simulink library "TQD_lib"  (Simulink 7.5)
settings: Solver=ode45  StartTime=0.0  StopTime=10.0  RelTol=1e-3
values from neighbouring files (symbols this model uses):
  pTQD_bool_ZeroCrossingEnabl_C = Simulink.Parameter    [TQD_par.m]
  pTQD_Nm_HiTqRecoverThd_C = Simulink.Parameter    [TQD_par.m]
  pTQD_Nm_MaxPrimTMTrq_C = Simulink.Parameter    [TQD_par.m]
  pTQD_Nm_MaxSecTMTrq_C = Simulink.Parameter    [TQD_par.m]
  pTQD_Nm_MinPrimTMTrq_C = Simulink.Parameter    [TQD_par.m]
  pTQD_Nm_MinSecTMTrq_C = Simulink.Parameter    [TQD_par.m]
  pTQD_Nm_TMTrqMinus_C = Simulink.Parameter    [TQD_par.m]
  pTQD_Nm_TqLowrCrossHiThd_C = Simulink.Parameter    [TQD_par.m]
  pTQD_Nm_TqLowrCrossThd_C = Simulink.Parameter    [TQD_par.m]
  pTQD_Nm_TqUpprCrossHiThd_C = Simulink.Parameter    [TQD_par.m]
  pTQD_Nm_TqUpprCrossThd_C = Simulink.Parameter    [TQD_par.m]
  pTQD_Nmps_TrqLoRateLimit_C = Simulink.Parameter    [TQD_par.m]
  pTQD_Nmps_TrqUpRateLimit_C = Simulink.Parameter    [TQD_par.m]
  pTQD_r_DrvNearZeroFilterFac_C = Simulink.Parameter    [TQD_par.m]
  pTQD_r_DrvZeroCrsFilterFac_C = Simulink.Parameter    [TQD_par.m]
  pTQD_r_NormalFilterFac_C = Simulink.Parameter    [TQD_par.m]
  pTQD_rpm_TMZeroSpd_C = Simulink.Parameter    [TQD_par.m]
  pTQD_s_TqZeroCrossTiout_C = Simulink.Parameter    [TQD_par.m]
undefined symbols (not defined in the file or in its folder): p_single_Minus_M, p_single_Plus_M, p_single_Zero_M, p_st_DrvModeFlg_C
libraries: BaseOperationLib_Browser x95, simulink x1
settings Model: Creator=wuaibin  LastModifiedBy=wuaibin

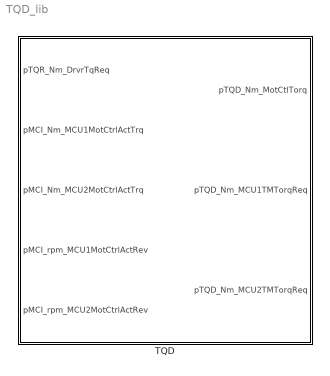
== system TQD_lib ==
  TQD : Subsystem  TreatAsAtomicUnit=on

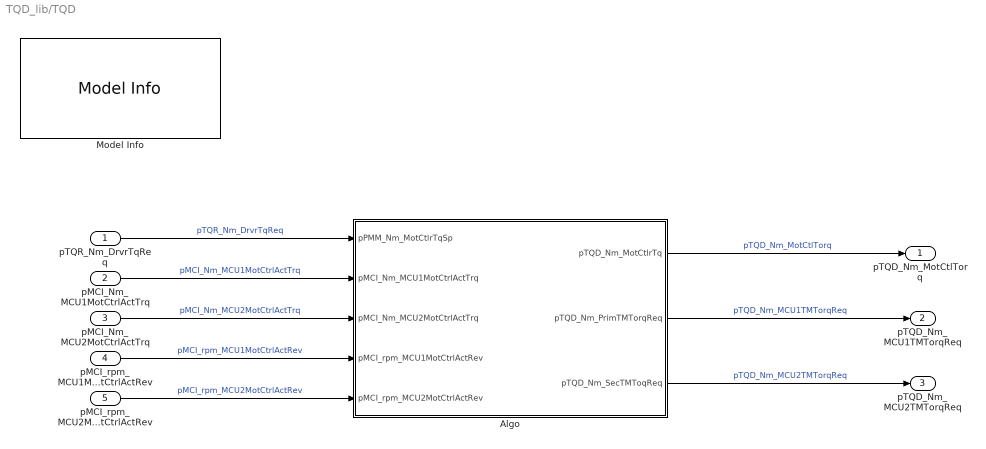
== system TQD_lib/TQD ==
  pTQR_Nm_DrvrTqReq : Inport  OutDataType=fixdt(1, 16)  OutScaling=2^0
  pMCI_Nm_MCU1MotCtrlActTrq : Inport  Port=2
  pMCI_Nm_MCU2MotCtrlActTrq : Inport  Port=3
  pMCI_rpm_MCU1MotCtrlActRev : Inport  Port=4  OutDataType=fixdt(1, 16)  OutScaling=2^0
  pMCI_rpm_MCU2MotCtrlActRev : Inport  Port=5  OutDataType=fixdt(1, 16)  OutScaling=2^0
  Algo : Subsystem
  Model Info : simulink/Model-Wide Utilities/Model Info  SystemSampleTime=-1  InitialBlockCM=None  BlockCM=None  Frame=on  DisplayStringWithTags=Model Info\nCreated: %<Created>\nCreator: %<Creator>  HorizontalTextAlignment=Center  LeftAlignmentValue=0.5  SourceBlockDiagram=HQEV_HCU  TagMaxNumber=20
  pTQD_Nm_MotCtlTorq : Outport  OutDataType=fixdt(1, 16)  OutScaling=2^0
  pTQD_Nm_MCU1TMTorqReq : Outport  Port=2
  pTQD_Nm_MCU2TMTorqReq : Outport  Port=3
  wires:
  pMCI_rpm_MCU2MotCtrlActRev/1 -> Algo/5(pMCI_rpm_MCU2MotCtrlActRev)  "pMCI_rpm_MCU2MotCtrlActRev"
  pMCI_rpm_MCU1MotCtrlActRev/1 -> Algo/4(pMCI_rpm_MCU1MotCtrlActRev)  "pMCI_rpm_MCU1MotCtrlActRev"
  pTQR_Nm_DrvrTqReq/1 -> Algo/1(pPMM_Nm_MotCtlrTqSp)  "pTQR_Nm_DrvrTqReq"
  pMCI_Nm_MCU1MotCtrlActTrq/1 -> Algo/2(pMCI_Nm_MCU1MotCtrlActTrq)  "pMCI_Nm_MCU1MotCtrlActTrq"
  pMCI_Nm_MCU2MotCtrlActTrq/1 -> Algo/3(pMCI_Nm_MCU2MotCtrlActTrq)  "pMCI_Nm_MCU2MotCtrlActTrq"
  Algo/1(pTQD_Nm_MotCtlrTq) -> pTQD_Nm_MotCtlTorq/1  "pTQD_Nm_MotCtlTorq"
  Algo/2(pTQD_Nm_PrimTMTorqReq) -> pTQD_Nm_MCU1TMTorqReq/1  "pTQD_Nm_MCU1TMTorqReq"
  Algo/3(pTQD_Nm_SecTMToqReq) -> pTQD_Nm_MCU2TMTorqReq/1  "pTQD_Nm_MCU2TMTorqReq"

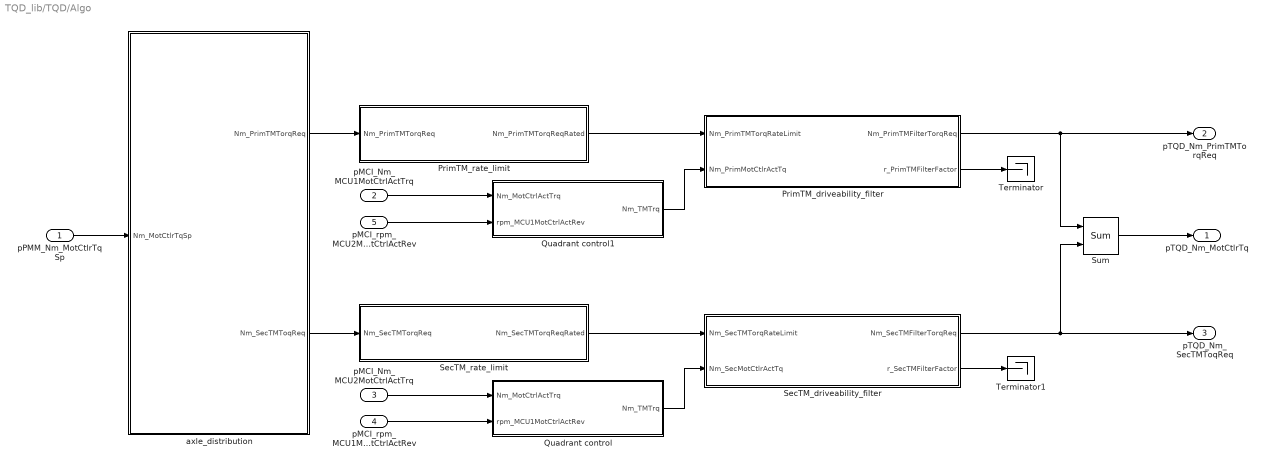
== system TQD_lib/TQD/Algo ==
  pPMM_Nm_MotCtlrTqSp : Inport  OutDataType=fixdt(1, 16)  OutScaling=2^0
  pMCI_Nm_MCU1MotCtrlActTrq : Inport  Port=2
  pMCI_Nm_MCU2MotCtrlActTrq : Inport  Port=3
  pMCI_rpm_MCU1MotCtrlActRev : Inport  Port=4  OutDataType=fixdt(1, 16)  OutScaling=2^0
  pMCI_rpm_MCU2MotCtrlActRev : Inport  Port=5  OutDataType=fixdt(1, 16)  OutScaling=2^0
  PrimTM_driveability_filter : Subsystem
  PrimTM_rate_limit : Subsystem
  Quadrant control : Subsystem
  Quadrant control1 : Subsystem
  SecTM_driveability_filter : Subsystem
  SecTM_rate_limit : Subsystem
  Sum : BaseOperationLib_Browser/Math Operations Changed/Sum  Inputs=++  InputSameDT=on  OutMin=[]  OutMax=[]  OutDataType=fixdt(1, 16)  OutScaling=2^0  SaturateOnIntegerOverflow=on
  Terminator : Terminator
  Terminator1 : Terminator
  axle_distribution : Subsystem
  pTQD_Nm_MotCtlrTq : Outport  OutDataType=fixdt(1, 16)  OutScaling=2^0
  pTQD_Nm_PrimTMTorqReq : Outport  Port=2
  pTQD_Nm_SecTMToqReq : Outport  Port=3
  wires:
  pMCI_rpm_MCU2MotCtrlActRev/1 -> Quadrant control1/2(rpm_MCU1MotCtrlActRev)
  pMCI_Nm_MCU1MotCtrlActTrq/1 -> Quadrant control1/1(Nm_MotCtrlActTrq)
  Quadrant control1/1(Nm_TMTrq) -> PrimTM_driveability_filter/2(Nm_PrimMotCtlrActTq)
  Quadrant control/1(Nm_TMTrq) -> SecTM_driveability_filter/2(Nm_SecMotCtlrActTq)
  pMCI_rpm_MCU1MotCtrlActRev/1 -> Quadrant control/2(rpm_MCU1MotCtrlActRev)
  pMCI_Nm_MCU2MotCtrlActTrq/1 -> Quadrant control/1(Nm_MotCtrlActTrq)
  SecTM_driveability_filter/1(Nm_SecTMFilterTorqReq) -> Sum/2, pTQD_Nm_SecTMToqReq/1
  PrimTM_driveability_filter/1(Nm_PrimTMFilterTorqReq) -> Sum/1, pTQD_Nm_PrimTMTorqReq/1
  pPMM_Nm_MotCtlrTqSp/1 -> axle_distribution/1(Nm_MotCtlrTqSp)
  Sum/1 -> pTQD_Nm_MotCtlrTq/1
  axle_distribution/1(Nm_PrimTMTorqReq) -> PrimTM_rate_limit/1(Nm_PrimTMTorqReq)
  PrimTM_rate_limit/1(Nm_PrimTMTorqReqRated) -> PrimTM_driveability_filter/1(Nm_PrimTMTorqRateLimit)
  SecTM_rate_limit/1(Nm_SecTMTorqReqRated) -> SecTM_driveability_filter/1(Nm_SecTMTorqRateLimit)
  axle_distribution/2(Nm_SecTMToqReq) -> SecTM_rate_limit/1(Nm_SecTMTorqReq)
  PrimTM_driveability_filter/2(r_PrimTMFilterFactor) -> Terminator/1
  SecTM_driveability_filter/2(r_SecTMFilterFactor) -> Terminator1/1

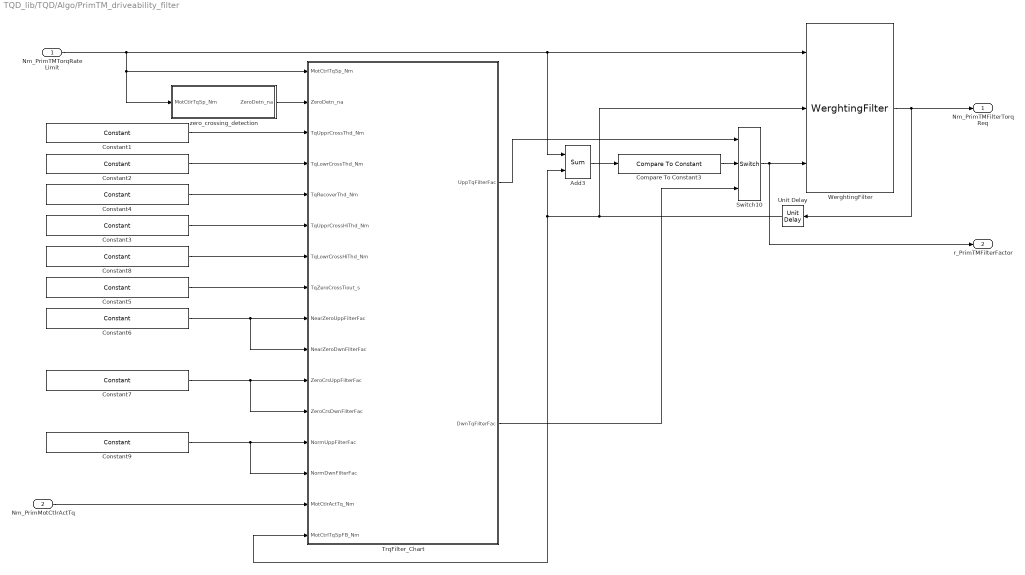
== system TQD_lib/TQD/Algo/PrimTM_driveability_filter ==
  Nm_PrimTMTorqRateLimit : Inport
  Nm_PrimMotCtlrActTq : Inport  Port=2
  Add3 : BaseOperationLib_Browser/Math Operations Changed/Sum  Inputs=+-  OutMin=[]  OutMax=[]  OutDataType=fixdt(1, 16)  OutScaling=2^0
  Compare To Constant3 : BaseOperationLib_Browser/Logic Operations Changed/Compare To Constant  SystemSampleTime=-1  relop=>=  const=p_single_Zero_M
  Constant1 : BaseOperationLib_Browser/Sources&Sinks/Constant  Value=pTQD_Nm_TqUpprCrossThd_C  OutMin=[]  OutMax=[]  OutDataType=fixdt(1, 16)  ConRadixGroup=Use specified scaling  OutScaling=2^0  OutDataTypeStr=Inherit: Inherit from 'Constant value'
  Constant2 : BaseOperationLib_Browser/Sources&Sinks/Constant  Value=pTQD_Nm_TqLowrCrossThd_C  OutMin=[]  OutMax=[]  OutDataType=fixdt(1, 16)  ConRadixGroup=Use specified scaling  OutScaling=2^0  OutDataTypeStr=Inherit: Inherit from 'Constant value'
  Constant3 : BaseOperationLib_Browser/Sources&Sinks/Constant  Value=pTQD_Nm_TqUpprCrossHiThd_C  OutMin=[]  OutMax=[]  OutDataType=fixdt(1, 16)  ConRadixGroup=Use specified scaling  OutScaling=2^0  OutDataTypeStr=Inherit: Inherit from 'Constant value'
  Constant4 : BaseOperationLib_Browser/Sources&Sinks/Constant  Value=pTQD_Nm_HiTqRecoverThd_C  OutMin=[]  OutMax=[]  OutDataType=fixdt(1, 16)  ConRadixGroup=Use specified scaling  OutScaling=2^0  OutDataTypeStr=Inherit: Inherit from 'Constant value'
  Constant5 : BaseOperationLib_Browser/Sources&Sinks/Constant  Value=pTQD_s_TqZeroCrossTiout_C  OutMin=[]  OutMax=[]  OutDataType=fixdt(1, 16)  ConRadixGroup=Use specified scaling  OutScaling=2^0  OutDataTypeStr=Inherit: Inherit from 'Constant value'
  Constant6 : BaseOperationLib_Browser/Sources&Sinks/Constant  Value=pTQD_r_DrvNearZeroFilterFac_C  OutMin=[]  OutMax=[]  OutDataType=fixdt(1, 16)  ConRadixGroup=Use specified scaling  OutScaling=2^0  OutDataTypeStr=Inherit: Inherit from 'Constant value'
  Constant7 : BaseOperationLib_Browser/Sources&Sinks/Constant  Value=pTQD_r_DrvZeroCrsFilterFac_C  OutMin=[]  OutMax=[]  OutDataType=fixdt(1, 16)  ConRadixGroup=Use specified scaling  OutScaling=2^0  OutDataTypeStr=Inherit: Inherit from 'Constant value'
  Constant8 : BaseOperationLib_Browser/Sources&Sinks/Constant  Value=pTQD_Nm_TqLowrCrossHiThd_C  OutMin=[]  OutMax=[]  OutDataType=fixdt(1, 16)  ConRadixGroup=Use specified scaling  OutScaling=2^0  OutDataTypeStr=Inherit: Inherit from 'Constant value'
  Constant9 : BaseOperationLib_Browser/Sources&Sinks/Constant  Value=pTQD_r_NormalFilterFac_C  OutMin=[]  OutMax=[]  OutDataTypeMode=single  OutDataType=fixdt(1, 16)  ConRadixGroup=Use specified scaling  OutScaling=2^0  OutDataTypeStr=single
  Switch10 : BaseOperationLib_Browser/Signal Routing Changed/Switch  Criteria=u2 ~= 0  Threshold=0  OutMin=[]  OutMax=[]  OutDataType=fixdt(1,16,0)  OutScaling=[]
  TrqFilter_Chart : Stateflow chart  TreatAsAtomicUnit=on
  Unit Delay : BaseOperationLib_Browser/Discrete Unchanged /Unit Delay  X0=0  SampleTime=-1
  WerghtingFilter : BaseOperationLib_Browser/Discontinuities Unchanged/WerghtingFilter  SystemSampleTime=-1
  zero_crossing_detection : Subsystem
  Nm_PrimTMFilterTorqReq : Outport
  r_PrimTMFilterFactor : Outport  Port=2
  wires:
  Nm_PrimMotCtlrActTq/1 -> TrqFilter_Chart/15(MotCtlrActTq_Nm)
  Nm_PrimTMTorqRateLimit/1 -> Add3/1, WerghtingFilter/1, zero_crossing_detection/1(MotCtlrTqSp_Nm), TrqFilter_Chart/1(MotCtrlTqSp_Nm)
  TrqFilter_Chart/1(UppTqFilterFac) -> Switch10/1
  WerghtingFilter/1 -> Nm_PrimTMFilterTorqReq/1, Unit Delay/1
  Unit Delay/1 -> WerghtingFilter/2, Add3/2, TrqFilter_Chart/16(MotCtrlTqSpFB_Nm)
  Add3/1 -> Compare To Constant3/1
  Compare To Constant3/1 -> Switch10/2
  Switch10/1 -> WerghtingFilter/3, r_PrimTMFilterFactor/1
  zero_crossing_detection/1(ZeroDetn_na) -> TrqFilter_Chart/2(ZeroDetn_na)
  Constant7/1 -> TrqFilter_Chart/11(ZeroCrsUppFilterFac), TrqFilter_Chart/12(ZeroCrsDwnFilterFac)
  TrqFilter_Chart/2(DwnTqFilterFac) -> Switch10/3
  Constant1/1 -> TrqFilter_Chart/3(TqUpprCrossThd_Nm)
  Constant2/1 -> TrqFilter_Chart/4(TqLowrCrossThd_Nm)
  Constant4/1 -> TrqFilter_Chart/5(TqRecoverThd_Nm)
  Constant3/1 -> TrqFilter_Chart/6(TqUpprCrossHiThd_Nm)
  Constant8/1 -> TrqFilter_Chart/7(TqLowrCrossHiThd_Nm)
  Constant5/1 -> TrqFilter_Chart/8(TqZeroCrossTiout_s)
  Constant6/1 -> TrqFilter_Chart/9(NearZeroUppFilterFac), TrqFilter_Chart/10(NearZeroDwnFilterFac)
  Constant9/1 -> TrqFilter_Chart/13(NormUppFilterFac), TrqFilter_Chart/14(NormDwnFilterFac)

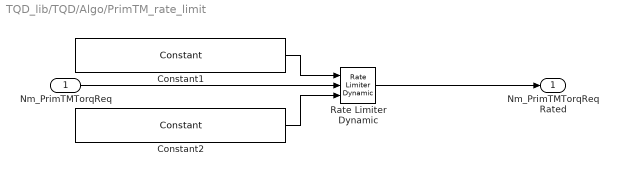
== system TQD_lib/TQD/Algo/PrimTM_rate_limit ==
  Nm_PrimTMTorqReq : Inport
  Constant1 : BaseOperationLib_Browser/Sources&Sinks/Constant  Value=pTQD_Nmps_TrqUpRateLimit_C  OutMin=[]  OutMax=[]  OutDataTypeMode=single  OutDataType=fixdt(1, 16)  ConRadixGroup=Use specified scaling  OutScaling=2^0  OutDataTypeStr=single
  Constant2 : BaseOperationLib_Browser/Sources&Sinks/Constant  Value=pTQD_Nmps_TrqLoRateLimit_C  OutMin=[]  OutMax=[]  OutDataTypeMode=single  OutDataType=fixdt(1, 16)  ConRadixGroup=Use specified scaling  OutScaling=2^0  OutDataTypeStr=single
  Rate Limiter Dynamic : BaseOperationLib_Browser/Discontinuities Unchanged/Rate Limiter Dynamic  SystemSampleTime=-1
  Nm_PrimTMTorqReqRated : Outport
  wires:
  Rate Limiter Dynamic/1 -> Nm_PrimTMTorqReqRated/1
  Nm_PrimTMTorqReq/1 -> Rate Limiter Dynamic/2
  Constant1/1 -> Rate Limiter Dynamic/1
  Constant2/1 -> Rate Limiter Dynamic/3

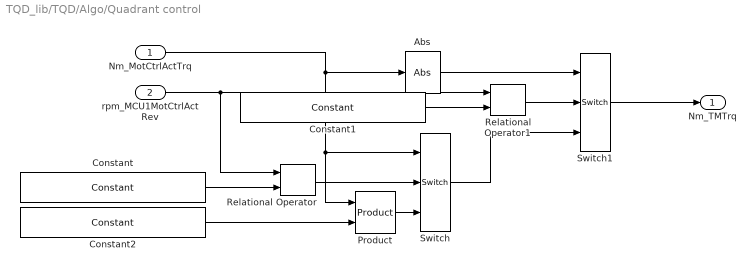
== system TQD_lib/TQD/Algo/Quadrant control ==
  Nm_MotCtrlActTrq : Inport
  rpm_MCU1MotCtrlActRev : Inport  Port=2  OutDataType=fixdt(1, 16)  OutScaling=2^0
  Abs : BaseOperationLib_Browser/Math Operations Changed/Abs  OutMax=[]  OutDataType=fixdt(1, 16)  OutScaling=2^0  SaturateOnIntegerOverflow=on
  Constant : BaseOperationLib_Browser/Sources&Sinks/Constant  Value=pTQD_rpm_TMZeroSpd_C  OutMin=[]  OutMax=[]  OutDataType=fixdt(1, 16)  ConRadixGroup=Use specified scaling  OutScaling=2^0  OutDataTypeStr=Inherit: Inherit from 'Constant value'
  Constant1 : BaseOperationLib_Browser/Sources&Sinks/Constant  Value=pTQD_rpm_TMZeroSpd_C  OutMin=[]  OutMax=[]  OutDataType=fixdt(1, 16)  ConRadixGroup=Use specified scaling  OutScaling=2^0  OutDataTypeStr=Inherit: Inherit from 'Constant value'
  Constant2 : BaseOperationLib_Browser/Sources&Sinks/Constant  Value=pTQD_Nm_TMTrqMinus_C  OutMin=[]  OutMax=[]  OutDataType=fixdt(1, 16)  ConRadixGroup=Use specified scaling  OutScaling=2^0  OutDataTypeStr=Inherit: Inherit from 'Constant value'
  Product : BaseOperationLib_Browser/Math Operations Changed/Product  Inputs=2  Multiplication=Element-wise(.*)  OutMin=[]  OutMax=[]  OutDataType=fixdt(1,16,0)  OutScaling=[]  OutDataTypeStr=Inherit: Inherit via back propagation  RndMeth=Zero  SaturateOnIntegerOverflow=on
  Relational Operator : BaseOperationLib_Browser/Logic Operations Changed/Relational Operator  Operator=>  InputSameDT=on  LogicOutDataTypeMode=Specify via dialog  LogicDataType=PDT_Bool  OutDataTypeStr=PDT_Bool
  Relational Operator1 : BaseOperationLib_Browser/Logic Operations Changed/Relational Operator  Operator===  InputSameDT=on  LogicOutDataTypeMode=Specify via dialog  LogicDataType=PDT_Bool  OutDataTypeStr=PDT_Bool
  Switch : BaseOperationLib_Browser/Signal Routing Changed/Switch  Criteria=u2 ~= 0  Threshold=1  InputSameDT=on  OutMin=[]  OutMax=[]  OutDataType=fixdt(1,16,0)  OutScaling=[]  SaturateOnIntegerOverflow=on
  Switch1 : BaseOperationLib_Browser/Signal Routing Changed/Switch  Criteria=u2 ~= 0  Threshold=1  InputSameDT=on  OutMin=[]  OutMax=[]  OutDataType=fixdt(1,16,0)  OutScaling=[]  SaturateOnIntegerOverflow=on
  Nm_TMTrq : Outport
  wires:
  Switch1/1 -> Nm_TMTrq/1
  rpm_MCU1MotCtrlActRev/1 -> Relational Operator/1, Relational Operator1/1
  Nm_MotCtrlActTrq/1 -> Product/1, Switch/1, Abs/1
  Constant2/1 -> Product/2
  Product/1 -> Switch/3
  Switch/1 -> Switch1/3
  Abs/1 -> Switch1/1
  Relational Operator1/1 -> Switch1/2
  Constant1/1 -> Relational Operator1/2
  Constant/1 -> Relational Operator/2
  Relational Operator/1 -> Switch/2

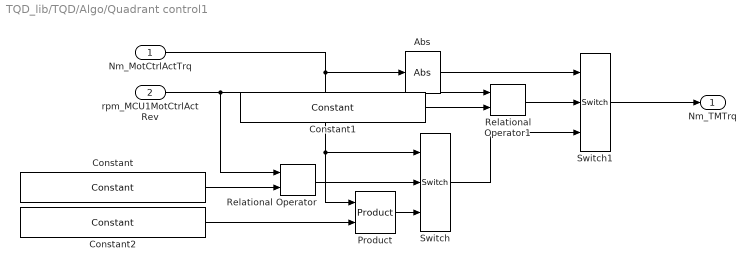
== system TQD_lib/TQD/Algo/Quadrant control1 ==
  Nm_MotCtrlActTrq : Inport
  rpm_MCU1MotCtrlActRev : Inport  Port=2  OutDataType=fixdt(1, 16)  OutScaling=2^0
  Abs : BaseOperationLib_Browser/Math Operations Changed/Abs  OutMax=[]  OutDataType=fixdt(1, 16)  OutScaling=2^0  SaturateOnIntegerOverflow=on
  Constant : BaseOperationLib_Browser/Sources&Sinks/Constant  Value=pTQD_rpm_TMZeroSpd_C  OutMin=[]  OutMax=[]  OutDataType=fixdt(1, 16)  ConRadixGroup=Use specified scaling  OutScaling=2^0  OutDataTypeStr=Inherit: Inherit from 'Constant value'
  Constant1 : BaseOperationLib_Browser/Sources&Sinks/Constant  Value=pTQD_rpm_TMZeroSpd_C  OutMin=[]  OutMax=[]  OutDataType=fixdt(1, 16)  ConRadixGroup=Use specified scaling  OutScaling=2^0  OutDataTypeStr=Inherit: Inherit from 'Constant value'
  Constant2 : BaseOperationLib_Browser/Sources&Sinks/Constant  Value=pTQD_Nm_TMTrqMinus_C  OutMin=[]  OutMax=[]  OutDataType=fixdt(1, 16)  ConRadixGroup=Use specified scaling  OutScaling=2^0  OutDataTypeStr=Inherit: Inherit from 'Constant value'
  Product : BaseOperationLib_Browser/Math Operations Changed/Product  Inputs=2  Multiplication=Element-wise(.*)  OutMin=[]  OutMax=[]  OutDataType=fixdt(1,16,0)  OutScaling=[]  OutDataTypeStr=Inherit: Inherit via back propagation  RndMeth=Zero  SaturateOnIntegerOverflow=on
  Relational Operator : BaseOperationLib_Browser/Logic Operations Changed/Relational Operator  Operator=>  InputSameDT=on  LogicOutDataTypeMode=Specify via dialog  LogicDataType=PDT_Bool  OutDataTypeStr=PDT_Bool
  Relational Operator1 : BaseOperationLib_Browser/Logic Operations Changed/Relational Operator  Operator===  InputSameDT=on  LogicOutDataTypeMode=Specify via dialog  LogicDataType=PDT_Bool  OutDataTypeStr=PDT_Bool
  Switch : BaseOperationLib_Browser/Signal Routing Changed/Switch  Criteria=u2 ~= 0  Threshold=1  InputSameDT=on  OutMin=[]  OutMax=[]  OutDataType=fixdt(1,16,0)  OutScaling=[]  SaturateOnIntegerOverflow=on
  Switch1 : BaseOperationLib_Browser/Signal Routing Changed/Switch  Criteria=u2 ~= 0  Threshold=1  InputSameDT=on  OutMin=[]  OutMax=[]  OutDataType=fixdt(1,16,0)  OutScaling=[]  SaturateOnIntegerOverflow=on
  Nm_TMTrq : Outport
  wires:
  Relational Operator/1 -> Switch/2
  Constant/1 -> Relational Operator/2
  Constant1/1 -> Relational Operator1/2
  Relational Operator1/1 -> Switch1/2
  Abs/1 -> Switch1/1
  Switch/1 -> Switch1/3
  Product/1 -> Switch/3
  Constant2/1 -> Product/2
  Nm_MotCtrlActTrq/1 -> Abs/1, Switch/1, Product/1
  rpm_MCU1MotCtrlActRev/1 -> Relational Operator1/1, Relational Operator/1
  Switch1/1 -> Nm_TMTrq/1

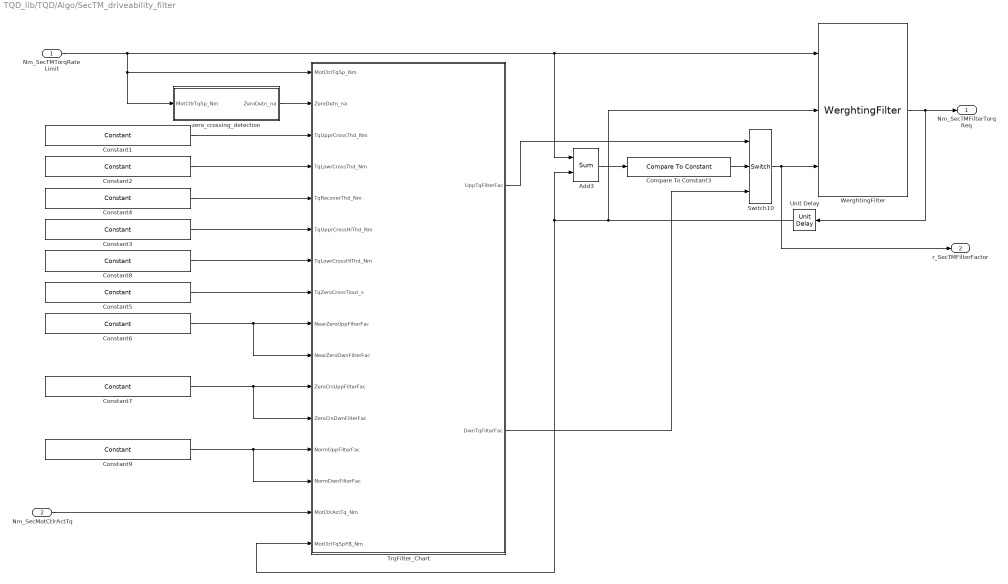
== system TQD_lib/TQD/Algo/SecTM_driveability_filter ==
  Nm_SecTMTorqRateLimit : Inport
  Nm_SecMotCtlrActTq : Inport  Port=2
  Add3 : BaseOperationLib_Browser/Math Operations Changed/Sum  Inputs=+-  OutMin=[]  OutMax=[]  OutDataType=fixdt(1, 16)  OutScaling=2^0
  Compare To Constant3 : BaseOperationLib_Browser/Logic Operations Changed/Compare To Constant  SystemSampleTime=-1  relop=>=  const=p_single_Zero_M
  Constant1 : BaseOperationLib_Browser/Sources&Sinks/Constant  Value=pTQD_Nm_TqUpprCrossThd_C  OutMin=[]  OutMax=[]  OutDataType=fixdt(1, 16)  ConRadixGroup=Use specified scaling  OutScaling=2^0  OutDataTypeStr=Inherit: Inherit from 'Constant value'
  Constant2 : BaseOperationLib_Browser/Sources&Sinks/Constant  Value=pTQD_Nm_TqLowrCrossThd_C  OutMin=[]  OutMax=[]  OutDataType=fixdt(1, 16)  ConRadixGroup=Use specified scaling  OutScaling=2^0  OutDataTypeStr=Inherit: Inherit from 'Constant value'
  Constant3 : BaseOperationLib_Browser/Sources&Sinks/Constant  Value=pTQD_Nm_TqUpprCrossHiThd_C  OutMin=[]  OutMax=[]  OutDataType=fixdt(1, 16)  ConRadixGroup=Use specified scaling  OutScaling=2^0  OutDataTypeStr=Inherit: Inherit from 'Constant value'
  Constant4 : BaseOperationLib_Browser/Sources&Sinks/Constant  Value=pTQD_Nm_HiTqRecoverThd_C  OutMin=[]  OutMax=[]  OutDataType=fixdt(1, 16)  ConRadixGroup=Use specified scaling  OutScaling=2^0  OutDataTypeStr=Inherit: Inherit from 'Constant value'
  Constant5 : BaseOperationLib_Browser/Sources&Sinks/Constant  Value=pTQD_s_TqZeroCrossTiout_C  OutMin=[]  OutMax=[]  OutDataType=fixdt(1, 16)  ConRadixGroup=Use specified scaling  OutScaling=2^0  OutDataTypeStr=Inherit: Inherit from 'Constant value'
  Constant6 : BaseOperationLib_Browser/Sources&Sinks/Constant  Value=pTQD_r_DrvNearZeroFilterFac_C  OutMin=[]  OutMax=[]  OutDataType=fixdt(1, 16)  ConRadixGroup=Use specified scaling  OutScaling=2^0  OutDataTypeStr=Inherit: Inherit from 'Constant value'
  Constant7 : BaseOperationLib_Browser/Sources&Sinks/Constant  Value=pTQD_r_DrvZeroCrsFilterFac_C  OutMin=[]  OutMax=[]  OutDataType=fixdt(1, 16)  ConRadixGroup=Use specified scaling  OutScaling=2^0  OutDataTypeStr=Inherit: Inherit from 'Constant value'
  Constant8 : BaseOperationLib_Browser/Sources&Sinks/Constant  Value=pTQD_Nm_TqLowrCrossHiThd_C  OutMin=[]  OutMax=[]  OutDataType=fixdt(1, 16)  ConRadixGroup=Use specified scaling  OutScaling=2^0  OutDataTypeStr=Inherit: Inherit from 'Constant value'
  Constant9 : BaseOperationLib_Browser/Sources&Sinks/Constant  Value=pTQD_r_NormalFilterFac_C  OutMin=[]  OutMax=[]  OutDataTypeMode=single  OutDataType=fixdt(1, 16)  ConRadixGroup=Use specified scaling  OutScaling=2^0  OutDataTypeStr=single
  Switch10 : BaseOperationLib_Browser/Signal Routing Changed/Switch  Criteria=u2 ~= 0  Threshold=0  OutMin=[]  OutMax=[]  OutDataType=fixdt(1,16,0)  OutScaling=[]
  TrqFilter_Chart : Stateflow chart  TreatAsAtomicUnit=on
  Unit Delay : BaseOperationLib_Browser/Discrete Unchanged /Unit Delay  X0=0  SampleTime=-1
  WerghtingFilter : BaseOperationLib_Browser/Discontinuities Unchanged/WerghtingFilter  SystemSampleTime=-1
  zero_crossing_detection : Subsystem
  Nm_SecTMFilterTorqReq : Outport
  r_SecTMFilterFactor : Outport  Port=2
  wires:
  Constant9/1 -> TrqFilter_Chart/14(NormDwnFilterFac), TrqFilter_Chart/13(NormUppFilterFac)
  Constant6/1 -> TrqFilter_Chart/10(NearZeroDwnFilterFac), TrqFilter_Chart/9(NearZeroUppFilterFac)
  Constant5/1 -> TrqFilter_Chart/8(TqZeroCrossTiout_s)
  Constant8/1 -> TrqFilter_Chart/7(TqLowrCrossHiThd_Nm)
  Constant3/1 -> TrqFilter_Chart/6(TqUpprCrossHiThd_Nm)
  Constant4/1 -> TrqFilter_Chart/5(TqRecoverThd_Nm)
  Constant2/1 -> TrqFilter_Chart/4(TqLowrCrossThd_Nm)
  Constant1/1 -> TrqFilter_Chart/3(TqUpprCrossThd_Nm)
  TrqFilter_Chart/2(DwnTqFilterFac) -> Switch10/3
  Constant7/1 -> TrqFilter_Chart/12(ZeroCrsDwnFilterFac), TrqFilter_Chart/11(ZeroCrsUppFilterFac)
  zero_crossing_detection/1(ZeroDetn_na) -> TrqFilter_Chart/2(ZeroDetn_na)
  Switch10/1 -> r_SecTMFilterFactor/1, WerghtingFilter/3
  Compare To Constant3/1 -> Switch10/2
  Add3/1 -> Compare To Constant3/1
  Unit Delay/1 -> TrqFilter_Chart/16(MotCtrlTqSpFB_Nm), Add3/2, WerghtingFilter/2
  WerghtingFilter/1 -> Unit Delay/1, Nm_SecTMFilterTorqReq/1
  TrqFilter_Chart/1(UppTqFilterFac) -> Switch10/1
  Nm_SecTMTorqRateLimit/1 -> TrqFilter_Chart/1(MotCtrlTqSp_Nm), zero_crossing_detection/1(MotCtlrTqSp_Nm), WerghtingFilter/1, Add3/1
  Nm_SecMotCtlrActTq/1 -> TrqFilter_Chart/15(MotCtlrActTq_Nm)

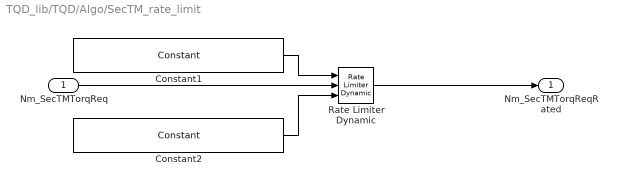
== system TQD_lib/TQD/Algo/SecTM_rate_limit ==
  Nm_SecTMTorqReq : Inport
  Constant1 : BaseOperationLib_Browser/Sources&Sinks/Constant  Value=pTQD_Nmps_TrqUpRateLimit_C  OutMin=[]  OutMax=[]  OutDataTypeMode=single  OutDataType=fixdt(1, 16)  ConRadixGroup=Use specified scaling  OutScaling=2^0  OutDataTypeStr=single
  Constant2 : BaseOperationLib_Browser/Sources&Sinks/Constant  Value=pTQD_Nmps_TrqLoRateLimit_C  OutMin=[]  OutMax=[]  OutDataTypeMode=single  OutDataType=fixdt(1, 16)  ConRadixGroup=Use specified scaling  OutScaling=2^0  OutDataTypeStr=single
  Rate Limiter Dynamic : BaseOperationLib_Browser/Discontinuities Unchanged/Rate Limiter Dynamic  SystemSampleTime=-1
  Nm_SecTMTorqReqRated : Outport
  wires:
  Constant2/1 -> Rate Limiter Dynamic/3
  Constant1/1 -> Rate Limiter Dynamic/1
  Nm_SecTMTorqReq/1 -> Rate Limiter Dynamic/2
  Rate Limiter Dynamic/1 -> Nm_SecTMTorqReqRated/1

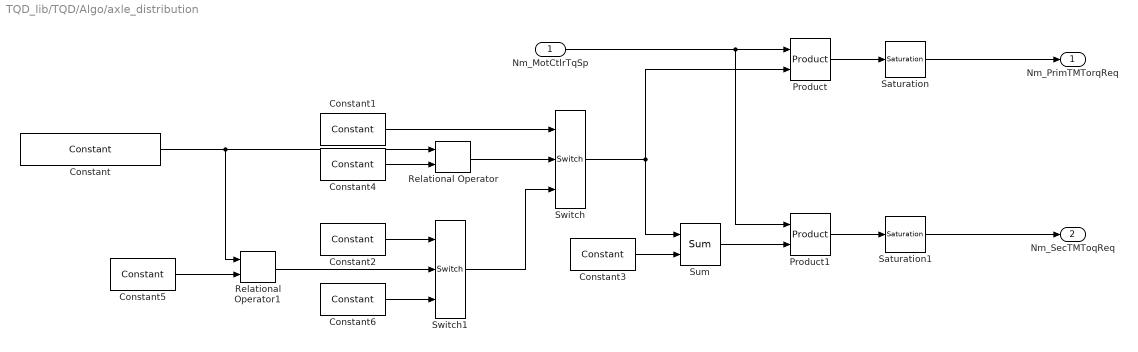
== system TQD_lib/TQD/Algo/axle_distribution ==
  Nm_MotCtlrTqSp : Inport
  Constant : BaseOperationLib_Browser/Sources&Sinks/Constant  Value=p_st_DrvModeFlg_C  OutMin=[]  OutMax=[]  OutDataType=fixdt(1, 16)  ConRadixGroup=Use specified scaling  OutScaling=2^0  OutDataTypeStr=Inherit: Inherit from 'Constant value'
  Constant1 : BaseOperationLib_Browser/Sources&Sinks/Constant  Value=1  OutMin=[]  OutMax=[]  OutDataTypeMode=single  OutDataType=fixdt(1, 16)  ConRadixGroup=Use specified scaling  OutScaling=2^0  OutDataTypeStr=single
  Constant2 : BaseOperationLib_Browser/Sources&Sinks/Constant  Value=0  OutMin=[]  OutMax=[]  OutDataTypeMode=single  OutDataType=fixdt(1, 16)  ConRadixGroup=Use specified scaling  OutScaling=2^0  OutDataTypeStr=single
  Constant3 : BaseOperationLib_Browser/Sources&Sinks/Constant  Value=1  OutMin=[]  OutMax=[]  OutDataTypeMode=single  OutDataType=fixdt(1, 16)  ConRadixGroup=Use specified scaling  OutScaling=2^0  OutDataTypeStr=single
  Constant4 : BaseOperationLib_Browser/Sources&Sinks/Constant  Value=1  OutMin=[]  OutMax=[]  OutDataTypeMode=uint8  OutDataType=fixdt(1, 16)  ConRadixGroup=Use specified scaling  OutScaling=2^0  OutDataTypeStr=uint8
  Constant5 : BaseOperationLib_Browser/Sources&Sinks/Constant  Value=2  OutMin=[]  OutMax=[]  OutDataTypeMode=uint8  OutDataType=fixdt(1, 16)  ConRadixGroup=Use specified scaling  OutScaling=2^0  OutDataTypeStr=uint8
  Constant6 : BaseOperationLib_Browser/Sources&Sinks/Constant  Value=0.5  OutMin=[]  OutMax=[]  OutDataTypeMode=single  OutDataType=fixdt(1, 16)  ConRadixGroup=Use specified scaling  OutScaling=2^0  OutDataTypeStr=single
  Product : BaseOperationLib_Browser/Math Operations Changed/Product  Inputs=2  Multiplication=Element-wise(.*)  OutMin=[]  OutMax=[]  OutDataType=fixdt(1,16,0)  OutScaling=[]  OutDataTypeStr=Inherit: Inherit via back propagation  RndMeth=Zero  SaturateOnIntegerOverflow=on
  Product1 : BaseOperationLib_Browser/Math Operations Changed/Product  Inputs=2  Multiplication=Element-wise(.*)  OutMin=[]  OutMax=[]  OutDataType=fixdt(1,16,0)  OutScaling=[]  OutDataTypeStr=Inherit: Inherit via back propagation  RndMeth=Zero  SaturateOnIntegerOverflow=on
  Relational Operator : BaseOperationLib_Browser/Logic Operations Changed/Relational Operator  Operator===  InputSameDT=on  LogicOutDataTypeMode=Specify via dialog  LogicDataType=PDT_Bool  OutDataTypeStr=PDT_Bool
  Relational Operator1 : BaseOperationLib_Browser/Logic Operations Changed/Relational Operator  Operator===  InputSameDT=on  LogicOutDataTypeMode=Specify via dialog  LogicDataType=PDT_Bool  OutDataTypeStr=PDT_Bool
  Saturation : BaseOperationLib_Browser/Discontinuities Unchanged/Saturation  UpperLimit=pTQD_Nm_MaxPrimTMTrq_C  LowerLimit=pTQD_Nm_MinPrimTMTrq_C  OutMin=[]  OutMax=[]  OutDataType=fixdt(1, 16)  OutScaling=2^0
      settings: AttributesFormatString=ULim:%<UpperLimit>\nLLim:%<LowerLimit>
  Saturation1 : BaseOperationLib_Browser/Discontinuities Unchanged/Saturation  UpperLimit=pTQD_Nm_MaxSecTMTrq_C  LowerLimit=pTQD_Nm_MinSecTMTrq_C  OutMin=[]  OutMax=[]  OutDataType=fixdt(1, 16)  OutScaling=2^0
      settings: AttributesFormatString=ULim:%<UpperLimit>\nLLim:%<LowerLimit>
  Sum : BaseOperationLib_Browser/Math Operations Changed/Sum  Inputs=-+  InputSameDT=on  OutMin=[]  OutMax=[]  OutDataType=fixdt(1, 16)  OutScaling=2^0  SaturateOnIntegerOverflow=on
  Switch : BaseOperationLib_Browser/Signal Routing Changed/Switch  Criteria=u2 ~= 0  Threshold=1  InputSameDT=on  OutMin=[]  OutMax=[]  OutDataType=fixdt(1,16,0)  OutScaling=[]  SaturateOnIntegerOverflow=on
  Switch1 : BaseOperationLib_Browser/Signal Routing Changed/Switch  Criteria=u2 ~= 0  Threshold=1  InputSameDT=on  OutMin=[]  OutMax=[]  OutDataType=fixdt(1,16,0)  OutScaling=[]  SaturateOnIntegerOverflow=on
  Nm_PrimTMTorqReq : Outport
  Nm_SecTMToqReq : Outport  Port=2
  wires:
  Saturation1/1 -> Nm_SecTMToqReq/1
  Product1/1 -> Saturation1/1
  Saturation/1 -> Nm_PrimTMTorqReq/1
  Product/1 -> Saturation/1
  Constant6/1 -> Switch1/3
  Constant2/1 -> Switch1/1
  Relational Operator1/1 -> Switch1/2
  Constant5/1 -> Relational Operator1/2
  Switch1/1 -> Switch/3
  Relational Operator/1 -> Switch/2
  Constant4/1 -> Relational Operator/2
  Constant/1 -> Relational Operator1/1, Relational Operator/1
  Nm_MotCtlrTqSp/1 -> Product1/1, Product/1
  Sum/1 -> Product1/2
  Constant3/1 -> Sum/2
  Switch/1 -> Sum/1, Product/2
  Constant1/1 -> Switch/1

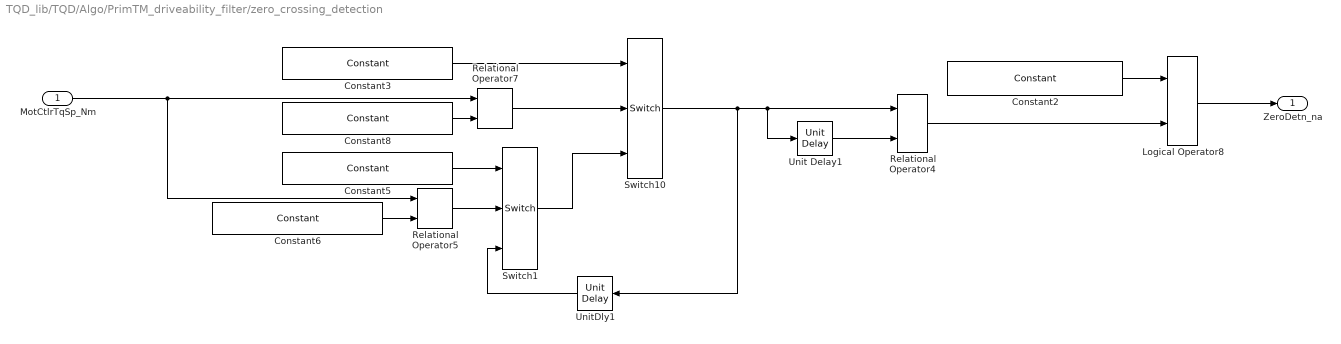
== system TQD_lib/TQD/Algo/PrimTM_driveability_filter/zero_crossing_detection ==
  MotCtlrTqSp_Nm : Inport
  Constant2 : BaseOperationLib_Browser/Sources&Sinks/Constant  Value=pTQD_bool_ZeroCrossingEnabl_C  OutMin=[]  OutMax=[]  OutDataType=fixdt(1, 16)  ConRadixGroup=Use specified scaling  OutScaling=2^0  OutDataTypeStr=Inherit: Inherit from 'Constant value'
  Constant3 : BaseOperationLib_Browser/Sources&Sinks/Constant  Value=p_single_Plus_M  OutMin=[]  OutMax=[]  OutDataType=fixdt(1, 16)  ConRadixGroup=Use specified scaling  OutScaling=2^0  OutDataTypeStr=Inherit: Inherit from 'Constant value'
  Constant5 : BaseOperationLib_Browser/Sources&Sinks/Constant  Value=p_single_Minus_M  OutMin=[]  OutMax=[]  OutDataType=fixdt(1, 16)  ConRadixGroup=Use specified scaling  OutScaling=2^0  OutDataTypeStr=Inherit: Inherit from 'Constant value'
  Constant6 : BaseOperationLib_Browser/Sources&Sinks/Constant  Value=p_single_Zero_M  OutMin=[]  OutMax=[]  OutDataType=fixdt(1, 16)  ConRadixGroup=Use specified scaling  OutScaling=2^0  OutDataTypeStr=Inherit: Inherit from 'Constant value'
  Constant8 : BaseOperationLib_Browser/Sources&Sinks/Constant  Value=p_single_Zero_M  OutMin=[]  OutMax=[]  OutDataType=fixdt(1, 16)  ConRadixGroup=Use specified scaling  OutScaling=2^0  OutDataTypeStr=Inherit: Inherit from 'Constant value'
  Logical Operator8 : BaseOperationLib_Browser/Logic Operations Changed/Logical Operator  Operator=AND  Inputs=2  AllPortsSameDT=off  OutDataTypeMode=boolean  LogicDataType=PDT_Bool  OutDataTypeStr=boolean
  Relational Operator4 : BaseOperationLib_Browser/Logic Operations Changed/Relational Operator  Operator=~=  InputSameDT=on  LogicOutDataTypeMode=Specify via dialog  LogicDataType=PDT_Bool  OutDataTypeStr=PDT_Bool
  Relational Operator5 : BaseOperationLib_Browser/Logic Operations Changed/Relational Operator  Operator=<  InputSameDT=on  LogicOutDataTypeMode=Specify via dialog  LogicDataType=PDT_Bool  OutDataTypeStr=PDT_Bool
  Relational Operator7 : BaseOperationLib_Browser/Logic Operations Changed/Relational Operator  Operator=>  InputSameDT=on  LogicOutDataTypeMode=Specify via dialog  LogicDataType=PDT_Bool  OutDataTypeStr=PDT_Bool
  Switch1 : BaseOperationLib_Browser/Signal Routing Changed/Switch  Criteria=u2 ~= 0  Threshold=0  OutMin=[]  OutMax=[]  OutDataType=fixdt(1,16,0)  OutScaling=[]
  Switch10 : BaseOperationLib_Browser/Signal Routing Changed/Switch  Criteria=u2 ~= 0  Threshold=0  OutMin=[]  OutMax=[]  OutDataType=fixdt(1,16,0)  OutScaling=[]
  Unit Delay1 : BaseOperationLib_Browser/Discrete Unchanged /Unit Delay  X0=0  SampleTime=-1
  UnitDly1 : BaseOperationLib_Browser/Discrete Unchanged /Unit Delay  X0=0  SampleTime=-1
  ZeroDetn_na : Outport
  wires:
  MotCtlrTqSp_Nm/1 -> Relational Operator7/1, Relational Operator5/1
  Unit Delay1/1 -> Relational Operator4/2
  Constant2/1 -> Logical Operator8/1
  Logical Operator8/1 -> ZeroDetn_na/1
  Constant8/1 -> Relational Operator7/2
  Relational Operator7/1 -> Switch10/2
  Switch10/1 -> UnitDly1/1, Relational Operator4/1, Unit Delay1/1
  Relational Operator5/1 -> Switch1/2
  Switch1/1 -> Switch10/3
  UnitDly1/1 -> Switch1/3
  Constant3/1 -> Switch10/1
  Constant6/1 -> Relational Operator5/2
  Constant5/1 -> Switch1/1
  Relational Operator4/1 -> Logical Operator8/2

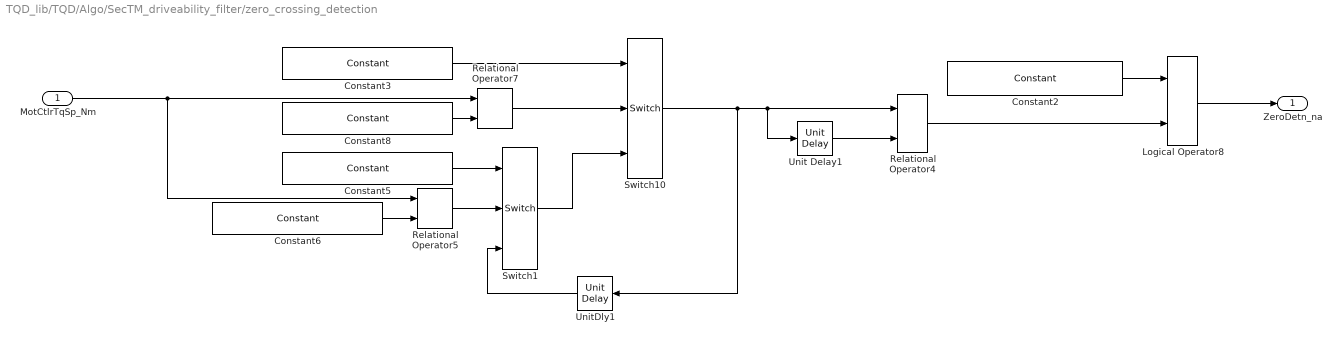
== system TQD_lib/TQD/Algo/SecTM_driveability_filter/zero_crossing_detection ==
  MotCtlrTqSp_Nm : Inport
  Constant2 : BaseOperationLib_Browser/Sources&Sinks/Constant  Value=pTQD_bool_ZeroCrossingEnabl_C  OutMin=[]  OutMax=[]  OutDataType=fixdt(1, 16)  ConRadixGroup=Use specified scaling  OutScaling=2^0  OutDataTypeStr=Inherit: Inherit from 'Constant value'
  Constant3 : BaseOperationLib_Browser/Sources&Sinks/Constant  Value=p_single_Plus_M  OutMin=[]  OutMax=[]  OutDataType=fixdt(1, 16)  ConRadixGroup=Use specified scaling  OutScaling=2^0  OutDataTypeStr=Inherit: Inherit from 'Constant value'
  Constant5 : BaseOperationLib_Browser/Sources&Sinks/Constant  Value=p_single_Minus_M  OutMin=[]  OutMax=[]  OutDataType=fixdt(1, 16)  ConRadixGroup=Use specified scaling  OutScaling=2^0  OutDataTypeStr=Inherit: Inherit from 'Constant value'
  Constant6 : BaseOperationLib_Browser/Sources&Sinks/Constant  Value=p_single_Zero_M  OutMin=[]  OutMax=[]  OutDataType=fixdt(1, 16)  ConRadixGroup=Use specified scaling  OutScaling=2^0  OutDataTypeStr=Inherit: Inherit from 'Constant value'
  Constant8 : BaseOperationLib_Browser/Sources&Sinks/Constant  Value=p_single_Zero_M  OutMin=[]  OutMax=[]  OutDataType=fixdt(1, 16)  ConRadixGroup=Use specified scaling  OutScaling=2^0  OutDataTypeStr=Inherit: Inherit from 'Constant value'
  Logical Operator8 : BaseOperationLib_Browser/Logic Operations Changed/Logical Operator  Operator=AND  Inputs=2  AllPortsSameDT=off  OutDataTypeMode=boolean  LogicDataType=PDT_Bool  OutDataTypeStr=boolean
  Relational Operator4 : BaseOperationLib_Browser/Logic Operations Changed/Relational Operator  Operator=~=  InputSameDT=on  LogicOutDataTypeMode=Specify via dialog  LogicDataType=PDT_Bool  OutDataTypeStr=PDT_Bool
  Relational Operator5 : BaseOperationLib_Browser/Logic Operations Changed/Relational Operator  Operator=<  InputSameDT=on  LogicOutDataTypeMode=Specify via dialog  LogicDataType=PDT_Bool  OutDataTypeStr=PDT_Bool
  Relational Operator7 : BaseOperationLib_Browser/Logic Operations Changed/Relational Operator  Operator=>  InputSameDT=on  LogicOutDataTypeMode=Specify via dialog  LogicDataType=PDT_Bool  OutDataTypeStr=PDT_Bool
  Switch1 : BaseOperationLib_Browser/Signal Routing Changed/Switch  Criteria=u2 ~= 0  Threshold=0  OutMin=[]  OutMax=[]  OutDataType=fixdt(1,16,0)  OutScaling=[]
  Switch10 : BaseOperationLib_Browser/Signal Routing Changed/Switch  Criteria=u2 ~= 0  Threshold=0  OutMin=[]  OutMax=[]  OutDataType=fixdt(1,16,0)  OutScaling=[]
  Unit Delay1 : BaseOperationLib_Browser/Discrete Unchanged /Unit Delay  X0=0  SampleTime=-1
  UnitDly1 : BaseOperationLib_Browser/Discrete Unchanged /Unit Delay  X0=0  SampleTime=-1
  ZeroDetn_na : Outport
  wires:
  Relational Operator4/1 -> Logical Operator8/2
  Constant5/1 -> Switch1/1
  Constant6/1 -> Relational Operator5/2
  Constant3/1 -> Switch10/1
  UnitDly1/1 -> Switch1/3
  Switch1/1 -> Switch10/3
  Relational Operator5/1 -> Switch1/2
  Switch10/1 -> Unit Delay1/1, Relational Operator4/1, UnitDly1/1
  Relational Operator7/1 -> Switch10/2
  Constant8/1 -> Relational Operator7/2
  Logical Operator8/1 -> ZeroDetn_na/1
  Constant2/1 -> Logical Operator8/1
  Unit Delay1/1 -> Relational Operator4/2
  MotCtlrTqSp_Nm/1 -> Relational Operator5/1, Relational Operator7/1

== stateflow chart TQD/Algo/PrimTM_driveability_filter/TrqFilter_Chart ==
  state TorqueNormalFilter
    en:
    UppTqFilterFac = NormUppFilterFac;
    DwnTqFilterFac = NormDwnFilterFac;
    RisingZeroDetn_na=false;
    FallingZeroDetn_na=false;
    du:
    UppTqFilterFac = NormUppFilterFac;
    DwnTqFilterFac = NormDwnFilterFac;
  state Driving
    state NearZeroFilter
      state NearZeroDwnFilter
        en:
        DwnTqFilterFac = NearZeroDwnFilterFac;
        du:
        DwnTqFilterFac = NearZeroDwnFilterFac;
      state NearZeroUppFilter
        en:
        UppTqFilterFac = NearZeroUppFilterFac;
        du:
        UppTqFilterFac = NearZeroUppFilterFac;
      (junction 12) -> NearZeroUppFilter [order 1] : [RisingZeroDetn_na == true]
      (junction 12) -> NearZeroDwnFilter [order 2]
      (default) -> (junction 12)
    state ZeroCrossingFilter
      state ZeroCrossingUppFilter
        en:
        UppTqFilterFac = ZeroCrsUppFilterFac;
        du:
        UppTqFilterFac = ZeroCrsUppFilterFac;
      state ZeroCrossingDwnFilter
        en:
        DwnTqFilterFac = ZeroCrsDwnFilterFac;
        du:
        DwnTqFilterFac = ZeroCrsDwnFilterFac;
      (junction 11) -> ZeroCrossingDwnFilter [order 2]
      (default) -> (junction 11)
      (junction 11) -> ZeroCrossingUppFilter [order 1] : [RisingZeroDetn_na == true]
    NearZeroFilter -> ZeroCrossingFilter : [(RisingZeroDetn_na&&MotCtlrActTq_Nm>= TqUpprCrossThd_Nm)|| ...
        | (FallingZeroDetn_na&&MotCtlrActTq_Nm<= TqLowrCrossThd_Nm)]
    (default) -> NearZeroFilter
  (default) -> TorqueNormalFilter
  TorqueNormalFilter -> Driving [order 2] : [ZeroDetn_na&&(MotCtrlTqSp_Nm>0)]
      | {RisingZeroDetn_na=true;
      | FallingZeroDetn_na=false;}
  Driving -> TorqueNormalFilter : [(abs(MotCtrlTqSp_Nm-MotCtrlTqSpFB_Nm)<=TqRecoverThd_Nm)|| ...
      | (RisingZeroDetn_na&&MotCtlrActTq_Nm>= TqUpprCrossHiThd_Nm)|| ...
      | (FallingZeroDetn_na&&MotCtlrActTq_Nm<= TqLowrCrossHiThd_Nm)|| ...
      | (after(TqZeroCrossTiout_s,sec))]
  TorqueNormalFilter -> Driving [order 1] : [ZeroDetn_na&&(MotCtrlTqSp_Nm<0)]
      | {RisingZeroDetn_na=false;
      | FallingZeroDetn_na=true;}
  data: MotCtrlTqSp_Nm input double; ZeroDetn_na input double; FallingZeroDetn_na local boolean; UppTqFilterFac output single; TqUpprCrossThd_Nm input double; TqLowrCrossThd_Nm input double; TqRecoverThd_Nm input double; TqUpprCrossHiThd_Nm input double; TqLowrCrossHiThd_Nm input double; TqZeroCrossTiout_s input double; NearZeroUppFilterFac input double; NearZeroDwnFilterFac input double; ZeroCrsUppFilterFac input double; ZeroCrsDwnFilterFac input double; NormUppFilterFac input double; NormDwnFilterFac input double; MotCtlrActTq_Nm input double; MotCtrlTqSpFB_Nm input double; RisingZeroDetn_na local boolean; DwnTqFilterFac output single

== stateflow chart TQD/Algo/SecTM_driveability_filter/TrqFilter_Chart ==
  state TorqueNormalFilter
    en:
    UppTqFilterFac = NormUppFilterFac;
    DwnTqFilterFac = NormDwnFilterFac;
    RisingZeroDetn_na=false;
    FallingZeroDetn_na=false;
    du:
    UppTqFilterFac = NormUppFilterFac;
    DwnTqFilterFac = NormDwnFilterFac;
  state Driving
    state NearZeroFilter
      state NearZeroDwnFilter
        en:
        DwnTqFilterFac = NearZeroDwnFilterFac;
        du:
        DwnTqFilterFac = NearZeroDwnFilterFac;
      state NearZeroUppFilter
        en:
        UppTqFilterFac = NearZeroUppFilterFac;
        du:
        UppTqFilterFac = NearZeroUppFilterFac;
      (junction 56) -> NearZeroUppFilter [order 1] : [RisingZeroDetn_na == true]
      (junction 56) -> NearZeroDwnFilter [order 2]
      (default) -> (junction 56)
    state ZeroCrossingFilter
      state ZeroCrossingUppFilter
        en:
        UppTqFilterFac = ZeroCrsUppFilterFac;
        du:
        UppTqFilterFac = ZeroCrsUppFilterFac;
      state ZeroCrossingDwnFilter
        en:
        DwnTqFilterFac = ZeroCrsDwnFilterFac;
        du:
        DwnTqFilterFac = ZeroCrsDwnFilterFac;
      (junction 55) -> ZeroCrossingDwnFilter [order 2]
      (default) -> (junction 55)
      (junction 55) -> ZeroCrossingUppFilter [order 1] : [RisingZeroDetn_na == true]
    NearZeroFilter -> ZeroCrossingFilter : [(RisingZeroDetn_na&&MotCtlrActTq_Nm>= TqUpprCrossThd_Nm)|| ...
        | (FallingZeroDetn_na&&MotCtlrActTq_Nm<= TqLowrCrossThd_Nm)]
    (default) -> NearZeroFilter
  (default) -> TorqueNormalFilter
  TorqueNormalFilter -> Driving [order 2] : [ZeroDetn_na&&(MotCtrlTqSp_Nm>0)]
      | {RisingZeroDetn_na=true;
      | FallingZeroDetn_na=false;}
  Driving -> TorqueNormalFilter : [(abs(MotCtrlTqSp_Nm-MotCtrlTqSpFB_Nm)<=TqRecoverThd_Nm)|| ...
      | (RisingZeroDetn_na&&MotCtlrActTq_Nm>= TqUpprCrossHiThd_Nm)|| ...
      | (FallingZeroDetn_na&&MotCtlrActTq_Nm<= TqLowrCrossHiThd_Nm)|| ...
      | (after(TqZeroCrossTiout_s,sec))]
  TorqueNormalFilter -> Driving [order 1] : [ZeroDetn_na&&(MotCtrlTqSp_Nm<0)]
      | {RisingZeroDetn_na=false;
      | FallingZeroDetn_na=true;}
  data: MotCtrlTqSp_Nm input double; ZeroDetn_na input double; FallingZeroDetn_na local boolean; UppTqFilterFac output single; TqUpprCrossThd_Nm input double; TqLowrCrossThd_Nm input double; TqRecoverThd_Nm input double; TqUpprCrossHiThd_Nm input double; TqLowrCrossHiThd_Nm input double; TqZeroCrossTiout_s input double; NearZeroUppFilterFac input double; NearZeroDwnFilterFac input double; ZeroCrsUppFilterFac input double; ZeroCrsDwnFilterFac input double; NormUppFilterFac input double; NormDwnFilterFac input double; MotCtlrActTq_Nm input double; MotCtrlTqSpFB_Nm input double; RisingZeroDetn_na local boolean; DwnTqFilterFac output single
